simulink model "sampleModel1473_3_sub"  (R2023a)
settings: Solver=VariableStepAuto  StartTime=0.0  StopTime=10.0  RelTol=1e-3
libraries: hdlsllib x6, simulink x1
settings Model: Creator=user1  LastModifiedBy=user1

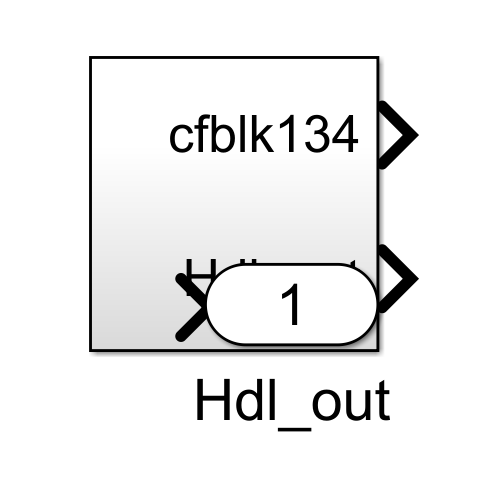
[thumbnail: Simulink's stored preview of the top-level diagram]
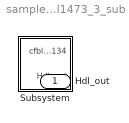
== system sampleModel1473_3_sub ==
  Subsystem : Subsystem
  Hdl_out : Outport  OutDataTypeStr=uint8

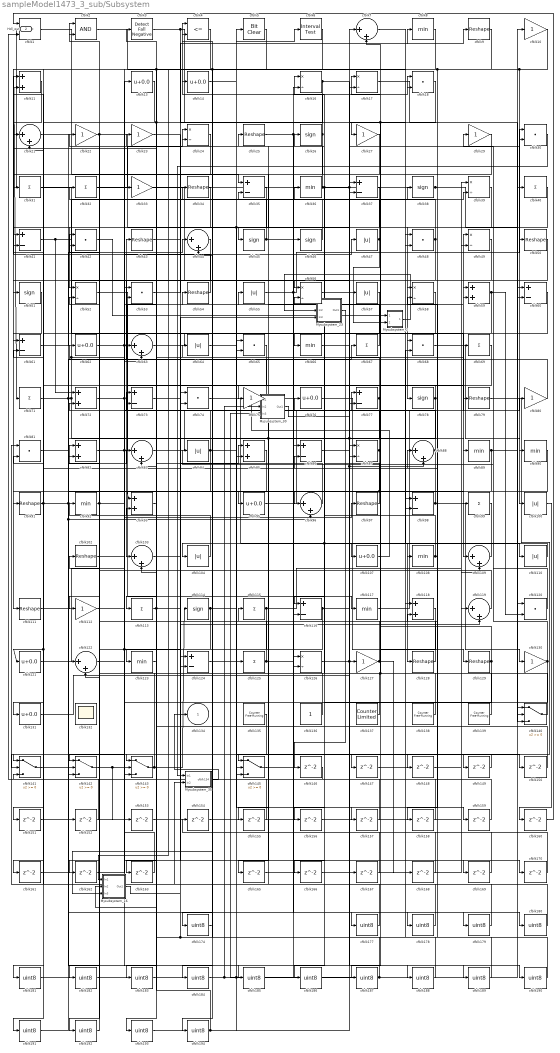
== system sampleModel1473_3_sub/Subsystem ==
  Mysubsystem_16 : Subsystem  TreatAsAtomicUnit=on  RTWFcnName=Mysubsystem_16
      settings: RTWFcnNameOpts=User specified  RTWFileNameOpts=Use function name
  Mysubsystem_2 : Subsystem  TreatAsAtomicUnit=on  RTWFcnName=Mysubsystem_2
      settings: RTWFcnNameOpts=User specified  RTWFileNameOpts=Use function name
  Mysubsystem_23 : Subsystem  TreatAsAtomicUnit=on  RTWFcnName=Mysubsystem_23
      settings: RTWFcnNameOpts=User specified  RTWFileNameOpts=Use function name
  Mysubsystem_30 : Subsystem  TreatAsAtomicUnit=on  RTWFcnName=Mysubsystem_30
      settings: RTWFcnNameOpts=User specified  RTWFileNameOpts=Use function name
  Mysubsystem_35 : Subsystem  TreatAsAtomicUnit=on  RTWFcnName=Mysubsystem_35
      settings: RTWFcnNameOpts=User specified  RTWFileNameOpts=Use function name
  cfblk1 : RelationalOperator  Operator=<=  OutDataTypeStr=boolean  InputSameDT=off
  cfblk{10,22..23,27,29,33,75,80,112,127,130} (11 alike) : Gain  OutDataTypeStr=uint8
  cfblk{47,55,57,64,84,100,104,110} (8 alike) : Abs  OutDataTypeStr=uint8  SaturateOnIntegerOverflow=off
  cfblk{9,25,34,43,50,54,79,91,97,102,111,128..129} (13 alike) : Reshape
  cfblk{7,21,44,63,83,88,96,103,109,119,122} (11 alike) : Sum  Inputs=|++  OutDataTypeStr=uint8
  cfblk{13..14,62,76,95,107,121,131} (8 alike) : Bias  Bias=0.0  SaturateOnIntegerOverflow=off
  cfblk{8,36,66,89..90,92,108,117,123} (9 alike) : MinMax  OutDataTypeStr=uint8
  cfblk{11,59,72,82,85,93,118} (7 alike) : Sum  OutDataTypeStr=uint8
  cfblk{31..32,40,67,69,71,99,113,115,125} (10 alike) : Sum  Inputs=+  OutDataTypeStr=uint8
  cfblk{26,38,45..46,51,78,114} (7 alike) : Signum
  cfblk{35,37,41,60..61,73,77,86,98,116,124} (11 alike) : Sum  Inputs=+-  OutDataTypeStr=uint8
  cfblk{18,30,42,48,53,65,68,74,81,120} (10 alike) : DotProduct  OutDataTypeStr=uint8
  cfblk{16..17,24,39,49,52,56,58,87,126} (10 alike) : Product  Inputs=*/  OutDataTypeStr=uint8  RndMeth=Zero  SaturateOnIntegerOverflow=on
  cfblk132 : Scope
      settings: Floating=on
  cfblk135 : hdlsllib/Sources/Counter Free-Running  NumBits=16  tsamp=-1
  cfblk136 : Constant  OutDataTypeStr=uint8  SampleTime=-1
  cfblk137 : hdlsllib/Sources/Counter Limited  uplimit=7  tsamp=-1
  cfblk138 : hdlsllib/Sources/Counter Free-Running  NumBits=16  tsamp=-1
  cfblk139 : hdlsllib/Sources/Counter Free-Running  NumBits=16  tsamp=-1
  cfblk{140..143,145} (5 alike) : Switch  OutDataTypeStr=uint8  SaturateOnIntegerOverflow=off  InputSameDT=off
  cfblk{146..163,165..170} (24 alike) : Delay  SampleTime=1
  cfblk{174,177..194} (19 alike) : DataTypeConversion  OutDataTypeStr=uint8  SaturateOnIntegerOverflow=off  RndMeth=Floor
  cfblk2 : Logic  AllPortsSameDT=off  OutDataTypeStr=boolean
  cfblk3 : hdlsllib/Logic and Bit Operations/Detect Fall Negative  vinit=0  OutDataTypeStr=uint8
  cfblk4 : RelationalOperator  Operator=<=  OutDataTypeStr=boolean  InputSameDT=off
  cfblk5 : simulink/Logic and Bit Operations/Bit Clear  iBit=0
      settings: LibrarySourceBlock=|
      | hdlsllib/Logic and Bit
      | Operations/Bit Clear
  cfblk6 : hdlsllib/Logic and Bit Operations/Interval Test  IntervalClosedRight=on  uplimit=0.5  IntervalClosedLeft=on  lowlimit=-0.5  OutDataTypeStr=uint8
  cfblk134 : Outport  OutDataTypeStr=uint8  VectorParamsAs1DForOutWhenUnconnected=off
  Hdl_out : Outport  Port=2  OutDataTypeStr=uint8
  wires:
  cfblk76/1 -> cfblk129/1
  cfblk26/1 -> cfblk4/2, cfblk111/1
  cfblk110/1 -> cfblk104/1
  cfblk32/1 -> cfblk24/1
  cfblk1/1 -> cfblk35/1
  cfblk8/1 -> cfblk174/1, cfblk193/1, cfblk71/1
  cfblk80/1 -> cfblk43/1
  cfblk79/1 -> cfblk142/1
  cfblk72/1 -> cfblk177/1, cfblk13/1
  cfblk71/1 -> cfblk98/2, cfblk98/1, cfblk55/1, cfblk38/1
  cfblk52/1 -> cfblk117/1
  cfblk139/1 -> cfblk16/1, cfblk77/1
  cfblk39/1 -> cfblk78/1
  cfblk54/1 -> cfblk11/1
  cfblk63/1 -> cfblk68/1
  cfblk44/1 -> cfblk103/1
  cfblk96/1 -> cfblk22/1
  cfblk35/1 -> cfblk145/3, cfblk121/1, cfblk141/1
  cfblk29/1 -> cfblk45/1
  cfblk131/1 -> cfblk57/1
  cfblk2/1 -> cfblk48/1
  cfblk3/1 -> cfblk27/1, cfblk48/2
  cfblk14/1 -> cfblk8/1
  cfblk83/1 -> cfblk49/1
  cfblk11/1 -> cfblk31/1
  cfblk85/1 -> cfblk91/1
  cfblk136/1 -> cfblk102/1
  cfblk98/1 -> cfblk11/2, cfblk130/1
  cfblk88/1 -> cfblk86/2, cfblk17/1
  cfblk77/1 -> cfblk116/2, cfblk21/1
  cfblk75/1 -> cfblk62/1, cfblk95/1, cfblk59/2
  cfblk145/1 -> cfblk46/1
  cfblk10/1 -> cfblk143/2, cfblk100/1
  cfblk97/1 -> cfblk36/1, cfblk93/1
  cfblk59/1 -> cfblk120/2, cfblk131/1
  cfblk65/1 -> cfblk181/1
  cfblk50/1 -> cfblk107/1
  cfblk87/1 -> cfblk192/1, cfblk24/2
  cfblk5/1 -> cfblk194/1
  cfblk118/1 -> cfblk187/1
  cfblk56/1 -> cfblk149/1, cfblk88/2
  cfblk58/1 -> cfblk113/1
  cfblk95/1 -> cfblk80/1
  cfblk82/1 -> cfblk76/1, cfblk54/1
  cfblk62/1 -> cfblk74/2, cfblk140/3, cfblk124/2
  cfblk78/1 -> cfblk75/1, cfblk87/2, cfblk155/1, cfblk142/2
  cfblk24/1 -> cfblk142/3
  cfblk22/1 -> cfblk112/1, cfblk127/1
  cfblk57/1 -> cfblk66/1
  cfblk143/1 -> cfblk42/2, cfblk114/1
  cfblk104/1 -> cfblk92/1
  cfblk60/1 -> cfblk184/1
  cfblk67/1 -> cfblk25/1
  cfblk41/1 -> cfblk72/1, cfblk109/1
  cfblk142/1 -> cfblk189/1, cfblk153/1
  cfblk129/1 -> cfblk156/1, cfblk7/2
  cfblk25/1 -> cfblk18/1, Mysubsystem_23/1(In1)
  cfblk114/1 -> cfblk162/1, cfblk6/1
  cfblk141/1 -> cfblk83/1
  cfblk47/1 -> cfblk34/1, Mysubsystem_2/2(In2)
  cfblk122/1 -> cfblk190/1
  cfblk33/1 -> cfblk87/1
  cfblk51/1 -> cfblk61/1
  cfblk117/1 -> cfblk10/1
  cfblk135/1 -> cfblk145/1
  cfblk130/1 -> cfblk140/2, cfblk29/1
  cfblk123/1 -> cfblk73/1
  cfblk68/1 -> cfblk90/1
  cfblk102/1 -> cfblk59/1
  cfblk74/1 -> cfblk128/1
  cfblk128/1 -> cfblk63/1
  cfblk17/1 -> cfblk120/1
  cfblk55/1 -> cfblk180/1, cfblk30/1
  cfblk53/1 -> cfblk9/1
  cfblk34/1 -> cfblk52/1
  cfblk125/1 -> cfblk159/1, cfblk14/1
  cfblk13/1 -> cfblk51/1
  cfblk73/1 -> cfblk79/1
  cfblk89/1 -> cfblk126/2, cfblk40/1
  cfblk49/1 -> cfblk58/1
  cfblk126/1 -> cfblk188/1, cfblk30/2
  cfblk138/1 -> cfblk64/1
  cfblk61/1 -> cfblk44/1
  cfblk140/1 -> cfblk26/1
  cfblk113/1 -> cfblk85/1, Mysubsystem_16/2(In2)
  cfblk92/1 -> cfblk52/2, cfblk33/1
  cfblk40/1 -> cfblk143/1
  cfblk109/1 -> cfblk108/1
  cfblk93/1 -> cfblk73/2
  cfblk119/1 -> cfblk2/1
  cfblk9/1 -> cfblk183/1, cfblk158/1
  cfblk86/1 -> cfblk69/1
  cfblk23/1 -> cfblk56/1
  cfblk116/1 -> cfblk39/2, cfblk145/2
  cfblk91/1 -> cfblk41/2, cfblk67/1, cfblk96/2, cfblk143/3
  cfblk48/1 -> cfblk191/1, cfblk23/1
  cfblk121/1 -> cfblk97/1
  cfblk18/1 -> cfblk147/1, cfblk37/2
  cfblk16/1 -> cfblk77/2, cfblk21/2, cfblk123/1
  cfblk31/1 -> cfblk126/1
  cfblk90/1 -> cfblk96/1
  cfblk7/1 -> cfblk110/1
  cfblk111/1 -> cfblk47/1
  cfblk127/1 -> cfblk168/1, cfblk82/1
  cfblk103/1 -> cfblk119/2
  cfblk66/1 -> cfblk89/1
  cfblk84/1 -> cfblk151/1, cfblk150/1, cfblk42/1
  cfblk37/1 -> cfblk41/1
  cfblk38/1 -> Hdl_out/1, cfblk140/1
  cfblk120/1 -> cfblk84/1
  cfblk64/1 -> cfblk56/2
  cfblk137/1 -> cfblk82/2
  cfblk108/1 -> cfblk148/1, cfblk72/2
  cfblk45/1 -> cfblk4/1, cfblk99/1
  cfblk99/1 -> cfblk166/1, cfblk165/1
  cfblk36/1 -> cfblk3/1, cfblk116/1, cfblk179/1, cfblk18/2
  cfblk115/1 -> cfblk163/1, cfblk50/1
  cfblk46/1 -> cfblk32/1
  cfblk146/1 -> cfblk1/2
  cfblk147/1 -> cfblk49/2
  cfblk148/1 -> cfblk58/2
  cfblk149/1 -> cfblk141/2
  cfblk150/1 -> cfblk103/2
  cfblk151/1 -> cfblk85/2
  cfblk21/1 -> cfblk152/1
  cfblk152/1 -> cfblk141/3
  cfblk153/1 -> cfblk119/1
  cfblk154/1 -> cfblk37/1
  cfblk155/1 -> cfblk83/2
  cfblk156/1 -> cfblk68/2
  cfblk124/1 -> cfblk157/1
  cfblk157/1 -> cfblk74/1
  cfblk158/1 -> cfblk2/2
  cfblk159/1 -> cfblk61/2
  cfblk100/1 -> cfblk160/1
  cfblk160/1 -> cfblk1/1
  cfblk6/1 -> cfblk161/1
  cfblk162/1 -> cfblk63/2
  cfblk163/1 -> cfblk53/1
  cfblk165/1 -> cfblk39/1
  cfblk166/1 -> cfblk109/2
  cfblk167/1 -> cfblk86/1
  cfblk168/1 -> cfblk44/2
  cfblk112/1 -> cfblk169/1
  cfblk169/1 -> cfblk88/1
  cfblk43/1 -> cfblk170/1
  cfblk170/1 -> cfblk35/2
  cfblk81/1 -> cfblk178/1
  cfblk178/1 -> cfblk115/1
  cfblk179/1 -> cfblk81/1
  cfblk180/1 -> cfblk81/2
  cfblk181/1 -> cfblk125/1, cfblk167/1
  cfblk27/1 -> cfblk182/1
  cfblk182/1 -> cfblk65/1
  cfblk183/1 -> cfblk65/2
  cfblk184/1 -> cfblk16/2, Mysubsystem_30/2(In2)
  cfblk161/1 -> cfblk185/1
  cfblk185/1 -> cfblk60/1
  cfblk69/1 -> cfblk186/1
  cfblk186/1 -> cfblk60/2
  cfblk187/1 -> cfblk154/1, Mysubsystem_30/3(In3)
  cfblk188/1 -> cfblk118/1
  cfblk189/1 -> cfblk118/2
  cfblk190/1 -> cfblk124/1, cfblk53/2
  cfblk191/1 -> cfblk122/1
  cfblk192/1 -> cfblk122/2
  cfblk193/1 -> cfblk5/1
  cfblk194/1 -> cfblk93/2, cfblk17/2
  cfblk42/1 -> Mysubsystem_2/1(In1)
  cfblk4/1 -> Mysubsystem_16/1(In1)
  cfblk174/1 -> Mysubsystem_16/3(In3)
  Mysubsystem_2/1(Out1) -> Mysubsystem_23/2(In2)
  Mysubsystem_16/1(Out1) -> Mysubsystem_23/3(In3)
  Mysubsystem_23/1(Out1) -> cfblk146/1
  cfblk107/1 -> Mysubsystem_30/1(In1)
  Mysubsystem_30/1(Out1) -> cfblk7/1
  cfblk30/1 -> Mysubsystem_35/1(In1)
  cfblk177/1 -> Mysubsystem_35/2(In2)
  Mysubsystem_35/1(cfblk134) -> cfblk134/1

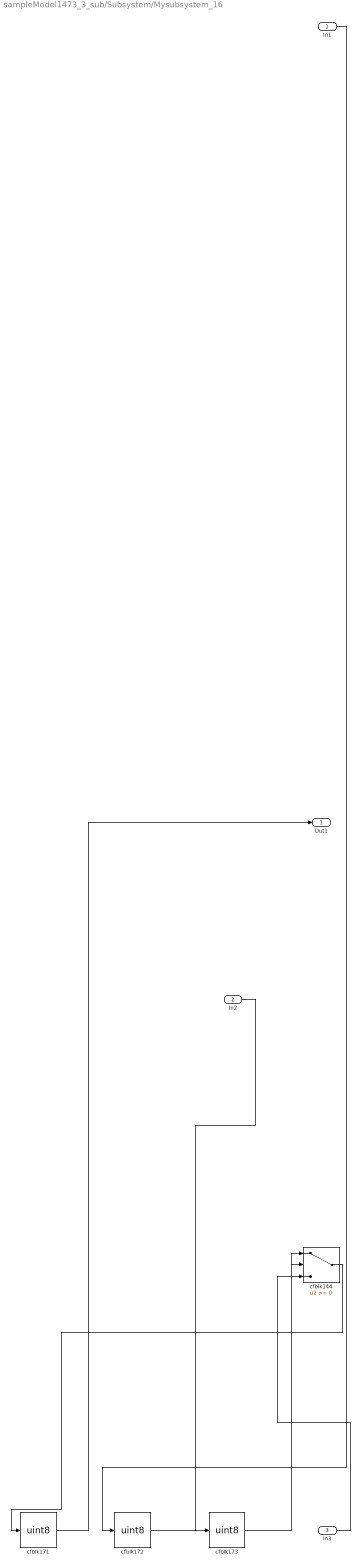
== system sampleModel1473_3_sub/Subsystem/Mysubsystem_16 ==
  In1 : Inport
  In2 : Inport  Port=2
  In3 : Inport  Port=3
  cfblk144 : Switch  SaturateOnIntegerOverflow=off  InputSameDT=off
  cfblk171 : DataTypeConversion  OutDataTypeStr=uint8  SaturateOnIntegerOverflow=off  RndMeth=Floor
  cfblk172 : DataTypeConversion  OutDataTypeStr=uint8  SaturateOnIntegerOverflow=off  RndMeth=Floor
  cfblk173 : DataTypeConversion  OutDataTypeStr=uint8  SaturateOnIntegerOverflow=off  RndMeth=Floor
  Out1 : Outport
  wires:
  In2/1 -> cfblk173/1
  cfblk171/1 -> Out1/1
  In1/1 -> cfblk172/1
  cfblk172/1 -> cfblk144/1
  cfblk144/1 -> cfblk171/1
  In3/1 -> cfblk144/3
  cfblk173/1 -> cfblk144/2

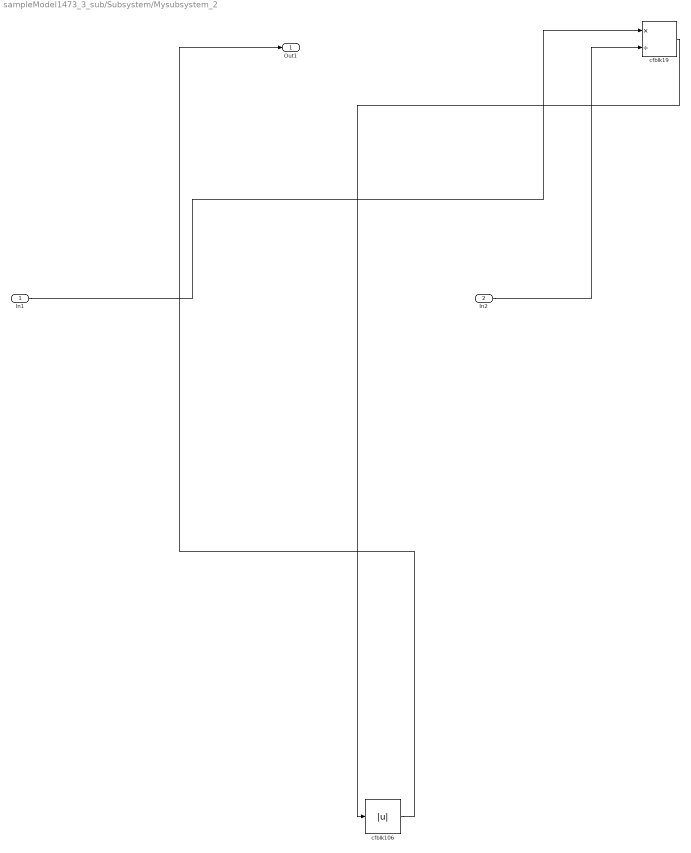
== system sampleModel1473_3_sub/Subsystem/Mysubsystem_2 ==
  In1 : Inport
  In2 : Inport  Port=2
  cfblk106 : Abs  SaturateOnIntegerOverflow=off
  cfblk19 : Product  Inputs=*/  RndMeth=Zero  SaturateOnIntegerOverflow=on
  Out1 : Outport
  wires:
  In1/1 -> cfblk19/1
  cfblk106/1 -> Out1/1
  cfblk19/1 -> cfblk106/1
  In2/1 -> cfblk19/2

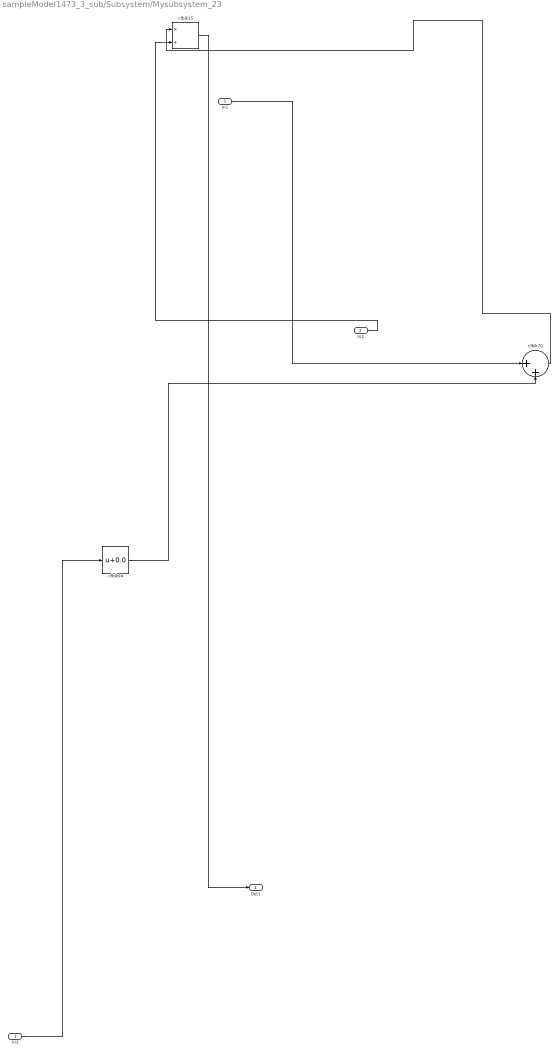
== system sampleModel1473_3_sub/Subsystem/Mysubsystem_23 ==
  In1 : Inport
  In2 : Inport  Port=2
  In3 : Inport  Port=3
  cfblk15 : Product  Inputs=*/  RndMeth=Zero  SaturateOnIntegerOverflow=on
  cfblk70 : Sum  Inputs=|++
  cfblk94 : Bias  Bias=0.0  SaturateOnIntegerOverflow=off
  Out1 : Outport
  wires:
  In1/1 -> cfblk70/1
  In3/1 -> cfblk94/1
  In2/1 -> cfblk15/2
  cfblk70/1 -> cfblk15/1
  cfblk94/1 -> cfblk70/2
  cfblk15/1 -> Out1/1

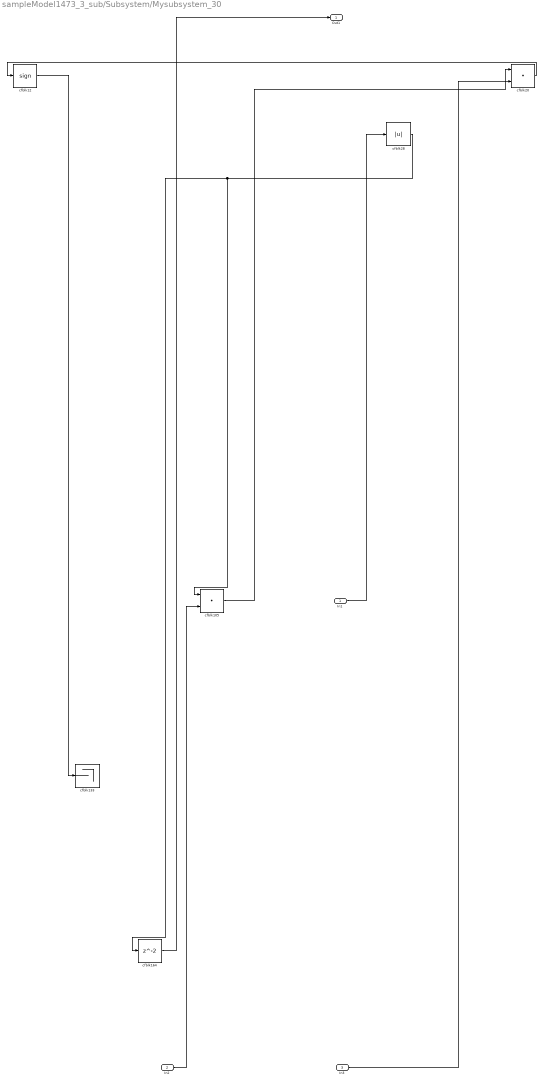
== system sampleModel1473_3_sub/Subsystem/Mysubsystem_30 ==
  In1 : Inport
  In2 : Inport  Port=2
  In3 : Inport  Port=3
  cfblk105 : DotProduct  OutDataTypeStr=Inherit: Inherit via internal rule
  cfblk12 : Signum
  cfblk133 : Terminator
  cfblk164 : Delay  SampleTime=1
  cfblk20 : DotProduct  OutDataTypeStr=Inherit: Inherit via internal rule
  cfblk28 : Abs  SaturateOnIntegerOverflow=off
  Out1 : Outport
  wires:
  In3/1 -> cfblk20/2
  In1/1 -> cfblk28/1
  cfblk105/1 -> cfblk20/1
  cfblk28/1 -> cfblk164/1, cfblk105/1
  In2/1 -> cfblk105/2
  cfblk164/1 -> Out1/1
  cfblk12/1 -> cfblk133/1
  cfblk20/1 -> cfblk12/1

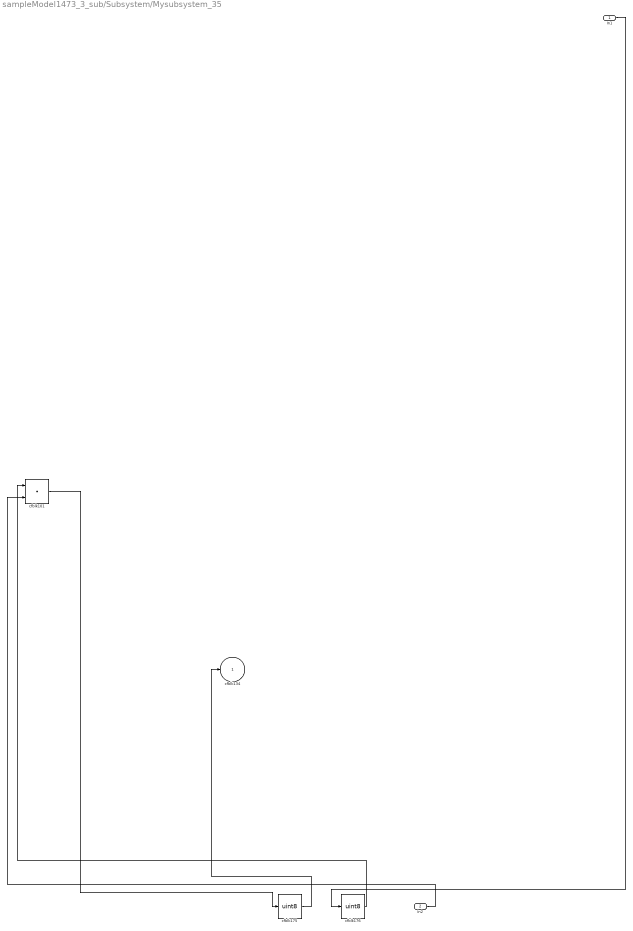
== system sampleModel1473_3_sub/Subsystem/Mysubsystem_35 ==
  In1 : Inport
  In2 : Inport  Port=2
  cfblk101 : DotProduct  OutDataTypeStr=Inherit: Inherit via internal rule
  cfblk175 : DataTypeConversion  OutDataTypeStr=uint8  SaturateOnIntegerOverflow=off  RndMeth=Floor
  cfblk176 : DataTypeConversion  OutDataTypeStr=uint8  SaturateOnIntegerOverflow=off  RndMeth=Floor
  cfblk134 : Outport  VectorParamsAs1DForOutWhenUnconnected=off
  wires:
  In1/1 -> cfblk176/1
  cfblk175/1 -> cfblk134/1
  cfblk176/1 -> cfblk101/1
  In2/1 -> cfblk101/2
  cfblk101/1 -> cfblk175/1
